simulink model "Homework3"  (R2024a)
settings: Solver=VariableStepAuto  StartTime=0.0  StopTime=25  FixedStep=0.1s  RelTol=1e-3
model workspace (MAT data in the model file):
  K = 500
undefined symbols (not defined in the file): den2_1, num2_1, tau_2
settings Model: Creator=Lxt10  LastModifiedBy=Lxt10

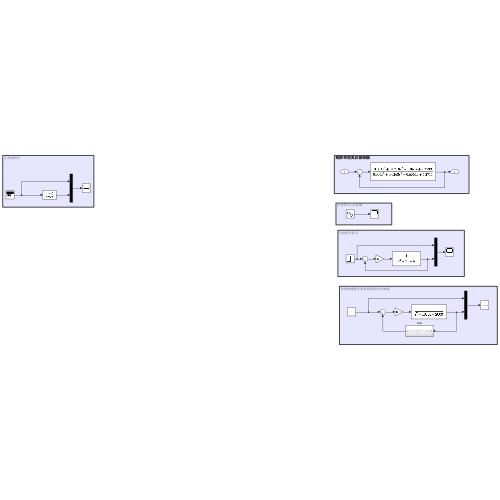
[thumbnail: Simulink's stored preview of the top-level diagram]
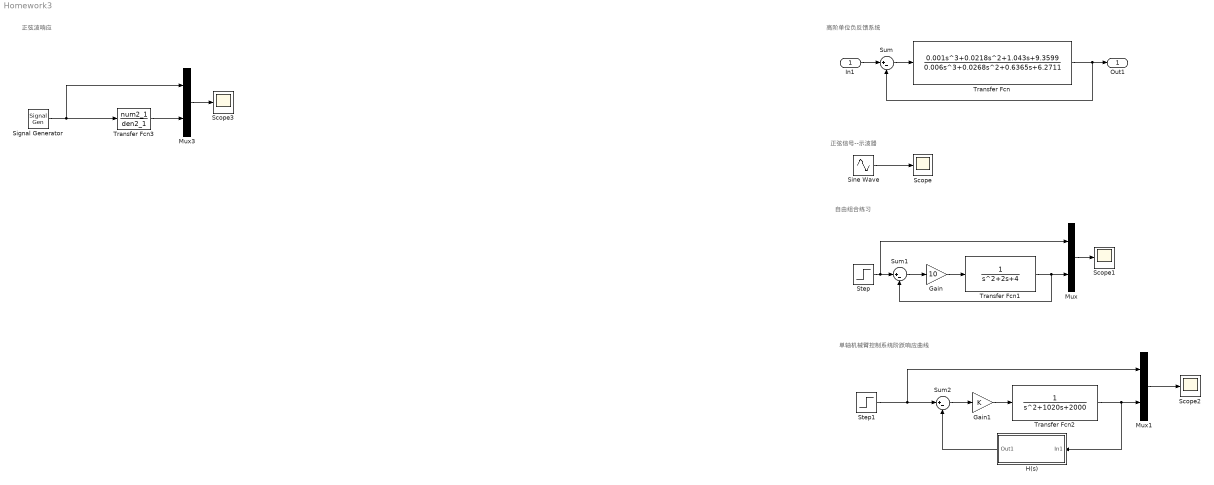
== system Homework3 ==
  note: 正弦波响应
  note: 单轴机械臂控制系统阶跃响应曲线
  note: 自由组合练习
  note: 正弦信号--示波器
  note: 高阶单位负反馈系统
  In1 : Inport
  Gain : Gain  Gain=10
  Gain1 : Gain  Gain=K
  H(s) : Subsystem
  Mux : Mux  Inputs=2
  Mux1 : Mux  Inputs=2
  Mux3 : Mux  Inputs=2
  Scope{,1..3} (4 alike) : Scope
  Signal Generator : SignalGenerator  Frequency=1/tau_2
  Sine Wave : Sin  SampleTime=0
  Step : Step  Time=5  After=10  SampleTime=0
  Step1 : Step  Time=5  SampleTime=0
  Sum : Sum  Inputs=|+-
  Sum1 : Sum  Inputs=|+-
  Sum2 : Sum  Inputs=|+-
  Transfer Fcn : TransferFcn  Numerator=[0.001 0.0218 1.043 9.3599]  Denominator=[0.006 0.0268 0.6365 6.2711]
  Transfer Fcn1 : TransferFcn  Denominator=[1 2 4]
  Transfer Fcn2 : TransferFcn  Denominator=[1 1020 2000]
  Transfer Fcn3 : TransferFcn  Numerator=num2_1  Denominator=den2_1
  Out1 : Outport
  wires:
  In1/1 -> Sum/1
  Sum/1 -> Transfer Fcn/1
  Transfer Fcn/1 -> Sum/2, Out1/1
  Sine Wave/1 -> Scope/1
  Gain/1 -> Transfer Fcn1/1
  Sum1/1 -> Gain/1
  Step/1 -> Mux/1, Sum1/1
  Transfer Fcn1/1 -> Mux/2, Sum1/2
  Mux/1 -> Scope1/1
  Step1/1 -> Mux1/1, Sum2/1
  Sum2/1 -> Gain1/1
  Gain1/1 -> Transfer Fcn2/1
  Transfer Fcn2/1 -> H(s)/1(In1), Mux1/2
  Mux1/1 -> Scope2/1
  H(s)/1(Out1) -> Sum2/2
  Transfer Fcn3/1 -> Mux3/2
  Mux3/1 -> Scope3/1
  Signal Generator/1 -> Transfer Fcn3/1, Mux3/1

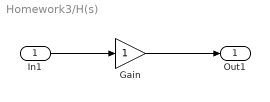
== system Homework3/H(s) ==
  In1 : Inport
  Gain : Gain
  Out1 : Outport
  wires:
  In1/1 -> Gain/1
  Gain/1 -> Out1/1
